simulink model "detect_threshold"  (R2014a)
settings: Solver=FixedStepDiscrete  StartTime=0.0  StopTime=10.0  RelTol=1e-3
InitFcn:
  | %% DSPBuilder Start
  | alt_dspbuilder_update_model(bdroot)
  | %% DSPBuilder End
model workspace (MAT data in the model file):
  Fs = 48000
libraries: simulink x5
settings Model: Creator=User  LastModifiedBy=User
settings OptimizationCC: InlineParams=on

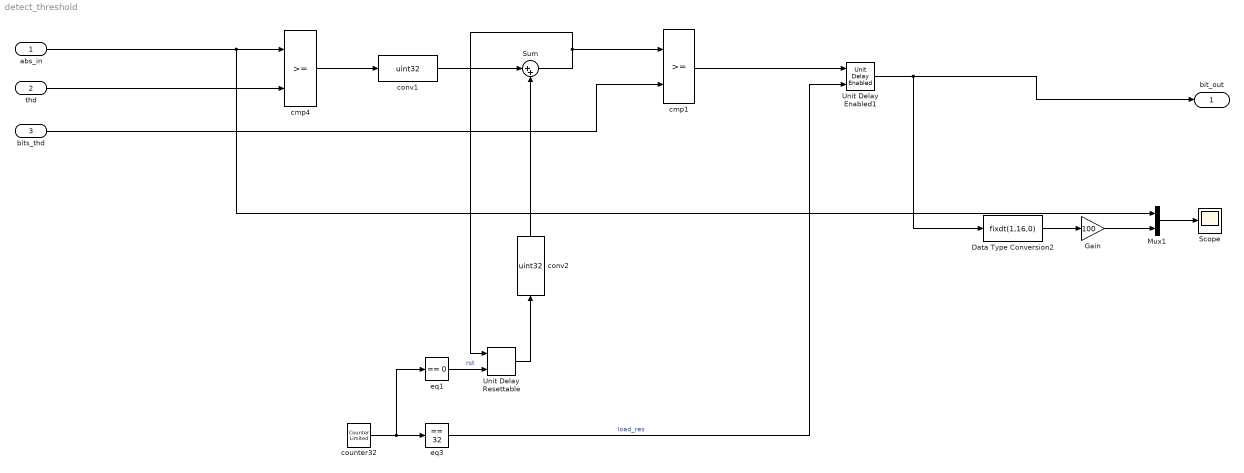
== system detect_threshold ==
  abs_in : Inport  OutDataTypeStr=fixdt(1,16,0)
  thd : Inport  Port=2  OutDataTypeStr=fixdt(1,16,0)
  bits_thd : Inport  Port=3  OutDataTypeStr=fixdt(1,16,0)
  Data Type Conversion2 : DataTypeConversion  OutDataTypeStr=fixdt(1,16,0)
  Gain : Gain  Gain=100  OutDataTypeStr=fixdt(1,16,0)
  Mux1 : Mux  Inputs=2
  Scope : Scope
      settings: YMin=0  YMax=750  MaxDataPoints=500000
  Sum : Sum  Inputs=|++
  Unit Delay Enabled1 : simulink/Additional Math & Discrete/Additional Discrete/Unit Delay Enabled  vinit=0.0  tsamp=-1
  Unit Delay Resettable : simulink/Additional Math & Discrete/Additional Discrete/Unit Delay Resettable  vinit=0.0  tsamp=-1
  cmp1 : RelationalOperator  OutDataTypeStr=boolean
  cmp4 : RelationalOperator  OutDataTypeStr=boolean
  conv1 : DataTypeConversion  OutDataTypeStr=uint32
  conv2 : DataTypeConversion  OutDataTypeStr=uint32
  counter32 : simulink/Sources/Counter Limited  uplimit=32  tsamp=-1
  eq1 : simulink/Logic and Bit Operations/Compare To Constant  relop===  const=0  OutDataTypeStr=boolean
  eq3 : simulink/Logic and Bit Operations/Compare To Constant  relop===  const=32  OutDataTypeStr=boolean
  bit_out : Outport
  wires:
  abs_in/1 -> Mux1/1, cmp4/1
  thd/1 -> cmp4/2
  counter32/1 -> eq1/1, eq3/1
  cmp4/1 -> conv1/1
  Mux1/1 -> Scope/1
  Sum/1 -> Unit Delay Resettable/1, cmp1/1
  Unit Delay Enabled1/1 -> Data Type Conversion2/1, bit_out/1
  eq3/1 -> Unit Delay Enabled1/2  "load_res"
  Unit Delay Resettable/1 -> conv2/1
  eq1/1 -> Unit Delay Resettable/2  "rst"
  cmp1/1 -> Unit Delay Enabled1/1
  conv1/1 -> Sum/1
  conv2/1 -> Sum/2
  Data Type Conversion2/1 -> Gain/1
  Gain/1 -> Mux1/2
  bits_thd/1 -> cmp1/2
